simulink model "BLDC_sims"  (R2024b)
settings: Solver=ode23s  StartTime=0.0  StopTime=3  MinStep=5e-5  RelTol=1e-3
values from neighbouring files (symbols this model uses):
  b_eq = b_l*(1/r)^2+b_m    (= 2.36823386114e-05)    [Parametros.m]
  c_pitch = cos(pitch)    [Parametros.m]
  J_eq = J_l*(1/r)^2+J_m    (= 7.12145792242e-06)    [Parametros.m]
  K_e = 0.0217    [Parametros.m]
  k_l = m*g*l_cm+m_l*g*l_l    (= 5.05042475)    [Parametros.m]
  K_t = 21.7e-3    (= 0.0217)    [Parametros.m]
  Kd_m = J_eq*n*w_pos    (= 0.0142429158448)    [Parametros.m]
  ke_int = w_obs^3    (= 125000000000)    [Parametros.m]
  ke_tita = w_obs*3    (= 15000)    [Parametros.m]
  ke_w = 3*w_obs^2    (= 75000000)    [Parametros.m]
  Ki_m = J_eq*w_pos^3    (= 3646.18645628)    [Parametros.m]
  Kp_m = J_eq*n*w_pos^2    (= 11.3943326759)    [Parametros.m]
  L_s = 0.113e-3    (= 0.000113)    [Parametros.m]
  p = 7    [Parametros.m]
  p_i = -3200    [Parametros.m]
  r = 156    [Parametros.m]
  R_s = 0.196    [Parametros.m]
  s_pitch = sin(pitch)    [Parametros.m]
  s_roll = sin(roll)    [Parametros.m]
  U_d = 18    [Parametros.m]
libraries: nesl_utility x17, ee_lib x13, fl_lib x9, sdl_lib x1, spsPWMGeneratorDCDCLib x1
settings Model: Creator=ribei  LastModifiedBy=ribei
settings DataIOCC: ExternalInput=q_vel  LoadExternalInput=on

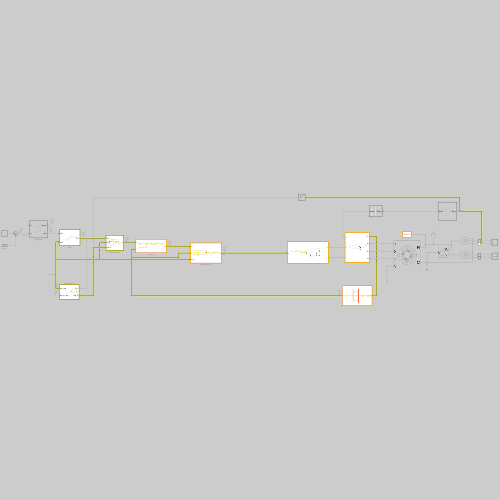
[thumbnail: Simulink's stored preview of the top-level diagram]
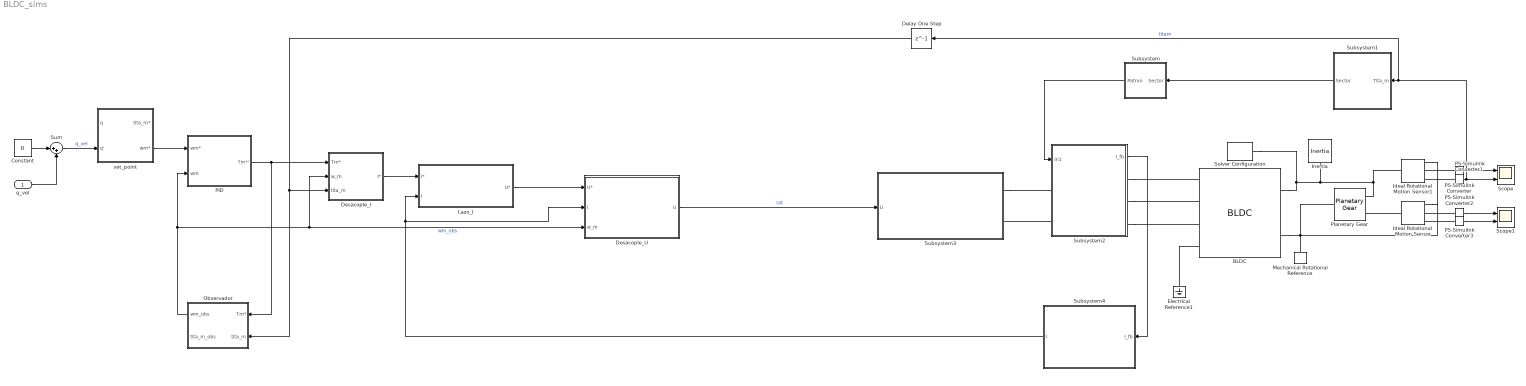
== system BLDC_sims ==
  q_vel : Inport
  BLDC : ee_lib/Electromechanical/Permanent Magnet/BLDC  port_option=ee.enum.threePhasePort.expanded  rotor_param=ee.enum.pmsm.backemf.trapezoidflux  pm_flux_linkage=0.0021 Wb  theta_constant=pi / 12 rad  emf_max=9.6 V  w_meas=600 rpm  DphiDtheta_tab=[0, -.1528, -.1528, .1528, .1528, 0] Wb/rad  back_emf_tab=[0, -9.6, -9.6, 9.6, 9.6, 0] V  rotor_angle_tab=[0, 7.5, 22.5, 37.5, 52.5, 60] deg  nPolePairs=7  axes_param=ee.enum.rotorangle.daxis  winding_type=ee.enum.electromech.statorconfiguration.wye  stator_param=ee.enum.statorparam.LdLqL0  machine_param=ee.enum.dqparameterization.constant  Ld=0.113 H  Lq=0.113 H  idVec=[-200, 0, 200] A  iqVec=[-200, 0, 200] A  LdMatrix=0.00022 * ones(3, 3) H  LqMatrix=0.00022 * ones(3, 3) H  L0=0.113 H  Ls=0.0002 H  Lm=0 H  Ms=0.00002 H  Rs=0.196 Ohm  zero_sequence=ee.enum.park.zerosequence.include  loss_param=ee.enum.ironloss.none  losses_oc=[0, 0, 0] W  losses_sc=[0, 0, 0] W  f_losses=60 Hz  Isc_losses=95 A  J=2.3e-6 kg*m^2  lam=1.184e-05 N*m*s/rad  i_d_specify=off  i_d_priority=None  i_d=0 A  i_d_nominal_specify=off  i_d_nominal_value=1  i_d_nominal_unit=A  i_q_specify=off  i_q_priority=None  i_q=0 A  i_q_nominal_specify=off  i_q_nominal_value=1  i_q_nominal_unit=A  torque_specify=off  torque_priority=None  torque=0 N*m  torque_nominal_specify=on  torque_nominal_value=0.105  torque_nominal_unit=N*m  angular_velocity_specify=off  angular_velocity_priority=High  angular_velocity=0 rpm  angular_velocity_nominal_specify=on  angular_velocity_nominal_value=6890  angular_velocity_nominal_unit=rpm  angular_position_specify=off  angular_position_priority=High  angular_position=0 deg  angular_position_nominal_specify=off  angular_position_nominal_value=1  angular_position_nominal_unit=deg  alpha=3.93e-3 1/K  alpha_flux=-0.001 1/K  Tmeas=298.15 K  stator_thermal_mass=100 J/K  rotor_thermal_mass=200 J/K  Rm_percent_rotor=90  Rd_percent_rotor=30  temperatureA_specify=off  temperatureA_priority=High  temperatureA=25 degC  temperatureA_nominal_specify=off  temperatureA_nominal_value=1  temperatureA_nominal_unit=degC  temperatureB_specify=off  temperatureB_priority=High  temperatureB=25 degC  temperatureB_nominal_specify=off  temperatureB_nominal_value=1  temperatureB_nominal_unit=degC  temperatureC_specify=off  temperatureC_priority=High  temperatureC=25 degC  temperatureC_nominal_specify=off  temperatureC_nominal_value=1  temperatureC_nominal_unit=degC  temperatureR_specify=off  temperatureR_priority=High  temperatureR=25 degC  temperatureR_nominal_specify=off  temperatureR_nominal_value=1  temperatureR_nominal_unit=degC
      settings: InternalSimscapePortConfiguration="{\"Bottom\":[],\"Left\":[{\"id\":\"a\",\"label\":\"a\",\"type\":\"foundation.electrical.electrical\"},{\"id\":\"b\",\"label\":\"b\",\"type\":\"foundation.electrical.electrical\"},{\"id\":\"c\",\"label\":\"c\",\"type\":\"foundation.electrical.electrical\"},{\"id\":\"n\",\"label\":\"n\",\"type\":\"foundation.electrical.electrical\"}],\"Right\":[{\"id\":\"R\",\"label\":\"R\",\"type\":\"foundation.mechanical.rotational.rotational\"},{\"id\":\"C\",\"label\":\"C\",\"type\":\"foundation.mechanical.rotational.rotational\"}],\"Top\":[]}"
  Constant : Constant  Value=0
  Delay One Step : Delay  DelayLength=1
  Desacople_I : Subsystem
  Desacople_U : Subsystem
  Electrical Reference1 : fl_lib/Electrical/Electrical Elements/Electrical Reference
  Ideal Rotational Motion Sensor : fl_lib/Mechanical/Mechanical Sensors/Ideal Rotational Motion Sensor  reference=foundation.enum.MeasurementReference.difference  acceleration_port=false  velocity_port=true  position_port=true  wrap_angle=false  offset=0 rad
  Ideal Rotational Motion Sensor1 : fl_lib/Mechanical/Mechanical Sensors/Ideal Rotational Motion Sensor  reference=foundation.enum.MeasurementReference.difference  acceleration_port=false  velocity_port=true  position_port=true  wrap_angle=false  offset=0 rad
  Inertia : fl_lib/Mechanical/Rotational Elements/Inertia  inertia=0.1173 kg*m^2  num_ports=foundation.enum.numPorts2.one  w_specify=off  w_priority=High  w=0 rad/s  w_nominal_specify=off  w_nominal_value=1  w_nominal_unit=rad/s  t_specify=off  t_priority=None  t=0 N*m  t_nominal_specify=off  t_nominal_value=1  t_nominal_unit=N*m
  Lazo_I : Subsystem
  Mechanical Rotational Reference : fl_lib/Mechanical/Rotational Elements/Mechanical Rotational Reference
  Observador : Subsystem
  PID : Subsystem
  PS-Simulink Converter{,1..3} (4 alike) : nesl_utility/PS-Simulink Converter  PhysicalDomain=network_engine_domain  SubClassName=ps_output  LeftPortType=input  RightPortType=output  PseudoPeriodic=off  Frequencies=[]  VectorFormat=inherit  Unit=inherit  AffineConversion=off
  Planetary Gear : sdl_lib/Gears/Planetary Gear  rs_ratio=156  friction_model=sdl.enum.gear_friction.none  efficiency=[.96, .98]  temperature_TLU=[280, 300, 320] K  efficiency_sp_TLU=[.95, .9, .85]  efficiency_rp_TLU=[.95, .9, .85]  pwr_thr=[.001, .001] W  mu_visc=[0, 0] N*m*s/rad  model_inertia=simscape.enum.onoff.off  sun_inertia=0.001 kg*m^2  ring_inertia=0.001 kg*m^2  carrier_inertia=0.001 kg*m^2  carrier_radius=0.01 m  planet_inertia=0.001 kg*m^2  planet_mass=0.001 kg  thermal_mass=50 J/K  T_init=300 K
  Scope : Scope  NumInputPorts=2
  Scope1 : Scope  NumInputPorts=2
  Solver Configuration : nesl_utility/Solver Configuration  PhysicalDomain=network_engine_domain  SubClassName=solver  LeftPortType=input  RightPortType=generic  Tones=[]  Harmonics=[]  SimulateNoise=off  Profile=off  UseLocalSampling=off  EnableSwitchedLinearOptims=on  FrequencyDomain=off  UseCCode=off  RelTol=0.001  AbsTol=0.001  MinStep=1e-09  ToWorkspace=off  RevertToSquareIcSolve=off  NumHomotopyIterations=100  PhasorMode=off  PhasorModeNumHarmonics=1  ConsistencySolver=NEWTON_XTOL_AFTER_FTOL  IndexReductionMethod=DerivativeReplacement  DoDC=off  ResidualTolerance=1e-09  ConsistencyTolSource=GLOBAL  ConsistencyAbsTol=0.001  ConsistencyRelTol=0.001  ConsistencyTolFactor=1e-9  UseLocalSolver=on  LocalSolverChoice=NE_BACKWARD_EULER_ADVANCER  ResolveIndetEquations=off  FunctionEvalNumThread=1  LocalSolverSampleTime=5e-5  DoFixedCost=on  MaxNonlinIter=3  MaxModeIter=2  ComputeImpulses=off  ImpulseIterations=2  LinearAlgebra=auto  LinearAlgebraNumThread=0  EquationFormulation=NE_TIME_EF  DelaysMemoryBudget=1024  AutomaticFiltering=on  FilteringTimeConstant=0.001  PartitionStorageMethod=AS_NEEDED  PartitionMemoryBudget=1024  PartitionMethod=ROBUST  MultibodyUseLocalSolver=off  MultibodyLocalSolverChoice=ODE1  MultibodyLocalSolverSampleTime=0.001
  Subsystem : Subsystem
  Subsystem1 : Subsystem
  Subsystem2 : Subsystem
  Subsystem3 : Subsystem
  Subsystem4 : Subsystem
  Sum : Sum  Inputs=|++
  set_point : Subsystem
  wires:
  Subsystem1/1(Sector) -> Subsystem/1(Sector)
  Subsystem/1(Patron) -> Subsystem2/1(In1)
  PS-Simulink Converter/1 -> Scope/1
  PS-Simulink Converter2/1 -> Scope1/1
  PS-Simulink Converter3/1 -> Scope1/2
  Subsystem4/1(I) -> Desacople_U/2(I), Lazo_I/2(I)
  Observador/1(wm_obs) -> PID/2(wm), Desacople_I/2(w_m), Desacople_U/3(w_m)  "wm_obs"
  PS-Simulink Converter1/1 -> Delay One Step/1, Subsystem1/1(Tita_m), Scope/2  "titam"
  set_point/2(wm*) -> PID/1(wm*)
  Lazo_I/1(U*) -> Desacople_U/1(U*)
  Constant/1 -> Sum/1
  Sum/1 -> set_point/2(q')  "q_vel"
  PID/1(Tm*') -> Observador/1(Tm*), Desacople_I/1(Tm*)
  q_vel/1 -> Sum/2
  Desacople_I/1(I*) -> Lazo_I/1(I*)
  Subsystem2/1(I_fb) -> Subsystem4/1(I_fb)
  Desacople_U/1(U) -> Subsystem3/1(U)  "Ud"
  Delay One Step/1 -> Observador/2(tita_m), Desacople_I/3(tita_m)
  connections:
  BLDC/RConn1 -- Solver Configuration/RConn1 -- Ideal Rotational Motion Sensor1/LConn1 -- Planetary Gear/RConn1 -- Inertia/LConn1
  BLDC/RConn2 -- Planetary Gear/LConn1 -- Mechanical Rotational Reference/LConn1 -- Ideal Rotational Motion Sensor1/RConn1 -- Ideal Rotational Motion Sensor/RConn1
  Ideal Rotational Motion Sensor/LConn1 -- Planetary Gear/RConn2
  PS-Simulink Converter/LConn1 -- Ideal Rotational Motion Sensor1/RConn2
  PS-Simulink Converter1/LConn1 -- Ideal Rotational Motion Sensor1/RConn3
  PS-Simulink Converter2/LConn1 -- Ideal Rotational Motion Sensor/RConn2
  PS-Simulink Converter3/LConn1 -- Ideal Rotational Motion Sensor/RConn3
  Subsystem2/RConn1 -- BLDC/LConn1
  Subsystem2/RConn2 -- BLDC/LConn2
  Subsystem2/RConn3 -- BLDC/LConn3
  Subsystem3/RConn1 -- Subsystem2/LConn1
  Subsystem2/LConn2 -- Subsystem3/RConn2
  BLDC/LConn4 -- Electrical Reference1/LConn1

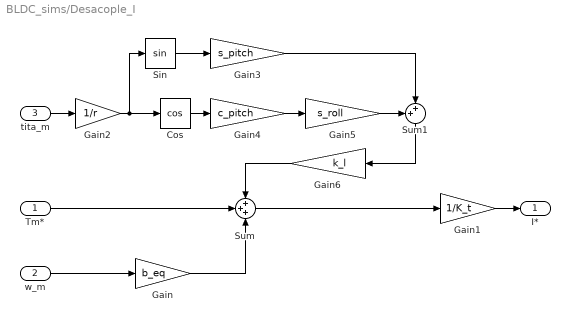
== system BLDC_sims/Desacople_I ==
  Tm* : Inport
  w_m : Inport  Port=2
  tita_m : Inport  Port=3
  Cos : Trigonometry  Operator=cos
  Gain : Gain  Gain=b_eq
  Gain1 : Gain  Gain=1/K_t
  Gain2 : Gain  Gain=1/r
  Gain3 : Gain  Gain=s_pitch
  Gain4 : Gain  Gain=c_pitch
  Gain5 : Gain  Gain=s_roll
  Gain6 : Gain  Gain=k_l
  Sin : Trigonometry
  Sum : Sum  Inputs=+++
  Sum1 : Sum  Inputs=++|
  I* : Outport
  wires:
  w_m/1 -> Gain/1
  Gain/1 -> Sum/3
  Sum/1 -> Gain1/1
  Gain1/1 -> I*/1
  Gain2/1 -> Cos/1, Sin/1
  tita_m/1 -> Gain2/1
  Cos/1 -> Gain4/1
  Sin/1 -> Gain3/1
  Sum1/1 -> Gain6/1
  Gain4/1 -> Gain5/1
  Gain5/1 -> Sum1/1
  Gain3/1 -> Sum1/2
  Gain6/1 -> Sum/1
  Tm*/1 -> Sum/2

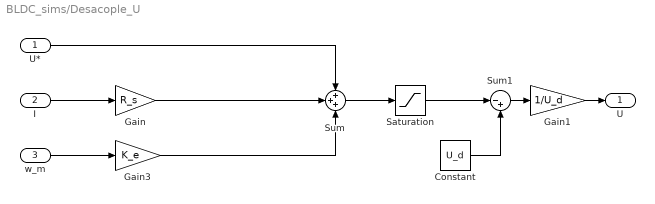
== system BLDC_sims/Desacople_U ==
  U* : Inport
  I : Inport  Port=2
  w_m : Inport  Port=3
  Constant : Constant  Value=U_d
  Gain : Gain  Gain=R_s
  Gain1 : Gain  Gain=1/U_d
  Gain3 : Gain  Gain=K_e
  Saturation : Saturate  UpperLimit=18  LowerLimit=-18
  Sum : Sum  Inputs=+++
  Sum1 : Sum  Inputs=|-+
  U : Outport
  wires:
  I/1 -> Gain/1
  w_m/1 -> Gain3/1
  Gain/1 -> Sum/2
  U*/1 -> Sum/1
  Gain3/1 -> Sum/3
  Sum/1 -> Saturation/1
  Saturation/1 -> Sum1/1
  Constant/1 -> Sum1/2
  Sum1/1 -> Gain1/1
  Gain1/1 -> U/1

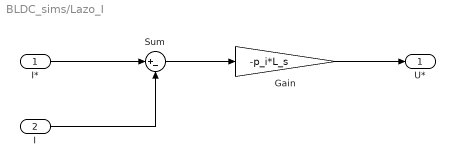
== system BLDC_sims/Lazo_I ==
  I* : Inport
  I : Inport  Port=2
  Gain : Gain  Gain=-p_i*L_s
  Sum : Sum  Inputs=|+-
  U* : Outport
  wires:
  I*/1 -> Sum/1
  I/1 -> Sum/2
  Gain/1 -> U*/1
  Sum/1 -> Gain/1

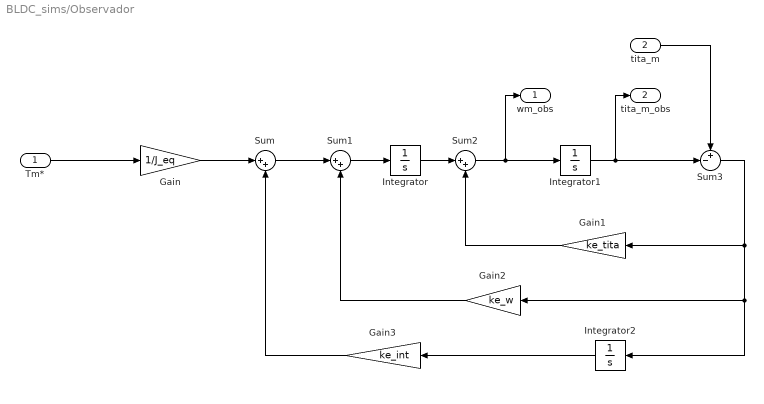
== system BLDC_sims/Observador ==
  Tm* : Inport
  tita_m : Inport  Port=2
  Gain : Gain  Gain=1/J_eq
  Gain1 : Gain  Gain=ke_tita
  Gain2 : Gain  Gain=ke_w
  Gain3 : Gain  Gain=ke_int
  Integrator : Integrator
  Integrator1 : Integrator  InitialCondition=pi/6
  Integrator2 : Integrator
  Sum : Sum  Inputs=|++
  Sum1 : Sum  Inputs=|++
  Sum2 : Sum  Inputs=|++
  Sum3 : Sum  Inputs=+-|
  wm_obs : Outport
  tita_m_obs : Outport  Port=2
  wires:
  Tm*/1 -> Gain/1
  Gain/1 -> Sum/1
  Sum/1 -> Sum1/1
  Sum1/1 -> Integrator/1
  Integrator/1 -> Sum2/1
  Sum2/1 -> wm_obs/1, Integrator1/1
  Integrator1/1 -> tita_m_obs/1, Sum3/2
  tita_m/1 -> Sum3/1
  Sum3/1 -> Gain1/1, Gain2/1, Integrator2/1
  Gain1/1 -> Sum2/2
  Gain2/1 -> Sum1/2
  Integrator2/1 -> Gain3/1
  Gain3/1 -> Sum/2

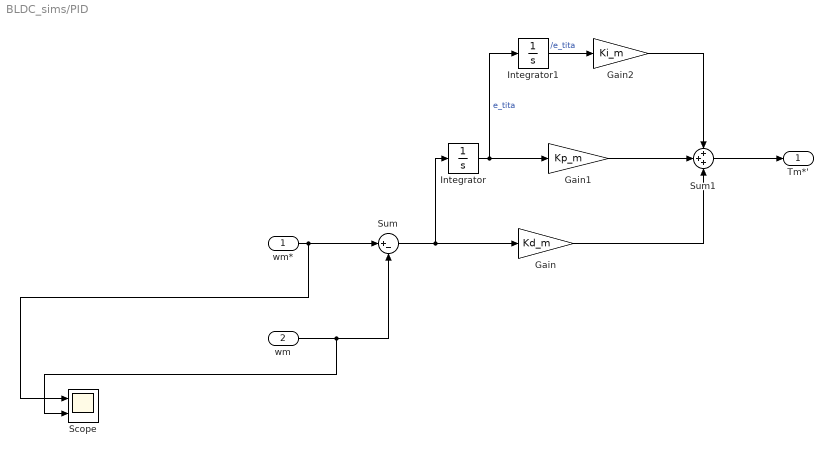
== system BLDC_sims/PID ==
  wm* : Inport
  wm : Inport  Port=2
  Gain : Gain  Gain=Kd_m
  Gain1 : Gain  Gain=Kp_m
  Gain2 : Gain  Gain=Ki_m
  Integrator : Integrator
  Integrator1 : Integrator
  Scope : Scope  NumInputPorts=2
  Sum : Sum  Inputs=|+-
  Sum1 : Sum  Inputs=+++
  Tm*' : Outport
  wires:
  Gain2/1 -> Sum1/1
  Gain/1 -> Sum1/3
  Gain1/1 -> Sum1/2
  Sum1/1 -> Tm*'/1
  wm/1 -> Scope/2, Sum/2
  Integrator/1 -> Gain1/1, Integrator1/1  "e_tita"
  Integrator1/1 -> Gain2/1  "/e_tita"
  wm*/1 -> Scope/1, Sum/1
  Sum/1 -> Gain/1, Integrator/1

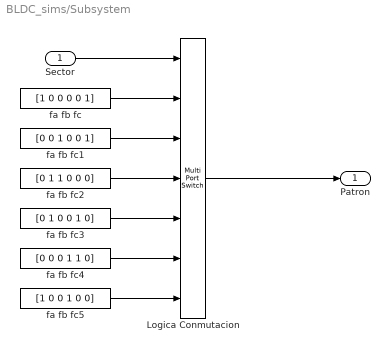
== system BLDC_sims/Subsystem ==
  Sector : Inport
  Logica Conmutacion : MultiPortSwitch  Inputs=6  DiagnosticForDefault=None  SaturateOnIntegerOverflow=off  InputSameDT=off
  fa fb fc : Constant  Value=[1 0 0 0 0 1]
  fa fb fc1 : Constant  Value=[0 0 1 0 0 1]
  fa fb fc2 : Constant  Value=[0 1 1 0 0 0]
  fa fb fc3 : Constant  Value=[0 1 0 0 1 0]
  fa fb fc4 : Constant  Value=[0 0 0 1 1 0]
  fa fb fc5 : Constant  Value=[1 0 0 1 0 0]
  Patron : Outport
  wires:
  fa fb fc3/1 -> Logica Conmutacion/5
  fa fb fc4/1 -> Logica Conmutacion/6
  fa fb fc1/1 -> Logica Conmutacion/3
  Sector/1 -> Logica Conmutacion/1
  Logica Conmutacion/1 -> Patron/1
  fa fb fc/1 -> Logica Conmutacion/2
  fa fb fc5/1 -> Logica Conmutacion/7
  fa fb fc2/1 -> Logica Conmutacion/4

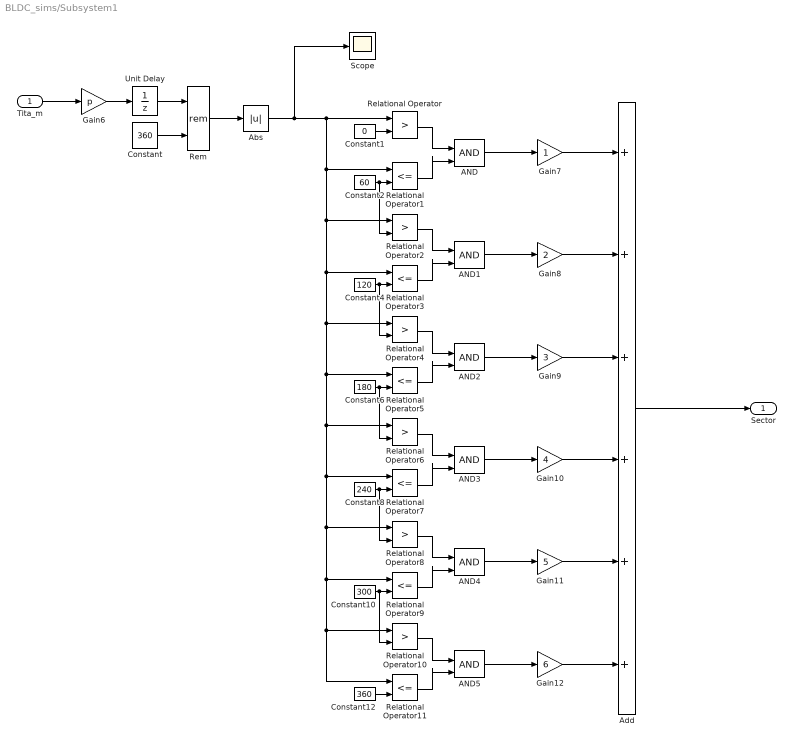
== system BLDC_sims/Subsystem1 ==
  Tita_m : Inport
  AND{,1..5} (6 alike) : Logic  IconShape=distinctive  AllPortsSameDT=off  OutDataTypeStr=boolean
  Abs : Abs  SaturateOnIntegerOverflow=off
  Add : Sum  Inputs=++++++
  Constant : Constant  Value=360
  Constant1 : Constant  Value=0
  Constant10 : Constant  Value=300
  Constant12 : Constant  Value=360
  Constant2 : Constant  Value=60
  Constant4 : Constant  Value=120
  Constant6 : Constant  Value=180
  Constant8 : Constant  Value=240
  Gain10 : Gain  Gain=4
  Gain11 : Gain  Gain=5
  Gain12 : Gain  Gain=6
  Gain6 : Gain  Gain=p
  Gain7 : Gain
  Gain8 : Gain  Gain=2
  Gain9 : Gain  Gain=3
  Relational Operator{,2,4,6,8,10} (6 alike) : RelationalOperator  Operator=>  OutDataTypeStr=boolean  RndMeth=Simplest  InputSameDT=off
  Relational Operator{1,3,5,7,9,11} (6 alike) : RelationalOperator  Operator=<=  OutDataTypeStr=boolean  RndMeth=Simplest  InputSameDT=off
  Rem : Math  Operator=rem
  Scope : Scope
  Unit Delay : UnitDelay  SampleTime=0.001  HasFrameUpgradeWarning=on
  Sector : Outport
  wires:
  Rem/1 -> Abs/1
  AND4/1 -> Gain11/1
  AND1/1 -> Gain8/1
  Relational Operator4/1 -> AND2/1
  Add/1 -> Sector/1
  Gain10/1 -> Add/4
  Relational Operator8/1 -> AND4/1
  Relational Operator3/1 -> AND1/2
  Relational Operator2/1 -> AND1/1
  Gain9/1 -> Add/3
  Constant4/1 -> Relational Operator4/2, Relational Operator3/2
  Constant6/1 -> Relational Operator6/2, Relational Operator5/2
  Gain11/1 -> Add/5
  Constant2/1 -> Relational Operator2/2, Relational Operator1/2
  AND2/1 -> Gain9/1
  Gain7/1 -> Add/1
  Relational Operator5/1 -> AND2/2
  Constant10/1 -> Relational Operator10/2, Relational Operator9/2
  AND/1 -> Gain7/1
  Constant1/1 -> Relational Operator/2
  Relational Operator/1 -> AND/1
  Constant/1 -> Rem/2
  Relational Operator11/1 -> AND5/2
  Constant12/1 -> Relational Operator11/2
  Relational Operator10/1 -> AND5/1
  AND5/1 -> Gain12/1
  Relational Operator9/1 -> AND4/2
  Unit Delay/1 -> Rem/1
  Gain12/1 -> Add/6
  Gain6/1 -> Unit Delay/1
  Tita_m/1 -> Gain6/1
  Constant8/1 -> Relational Operator8/2, Relational Operator7/2
  Relational Operator1/1 -> AND/2
  Relational Operator7/1 -> AND3/2
  AND3/1 -> Gain10/1
  Relational Operator6/1 -> AND3/1
  Gain8/1 -> Add/2
  Abs/1 -> Scope/1, Relational Operator/1, Relational Operator1/1, Relational Operator2/1, Relational Operator3/1, Relational Operator4/1, Relational Operator5/1, Relational Operator6/1, Relational Operator7/1, Relational Operator8/1, Relational Operator9/1, Relational Operator10/1, Relational Operator11/1

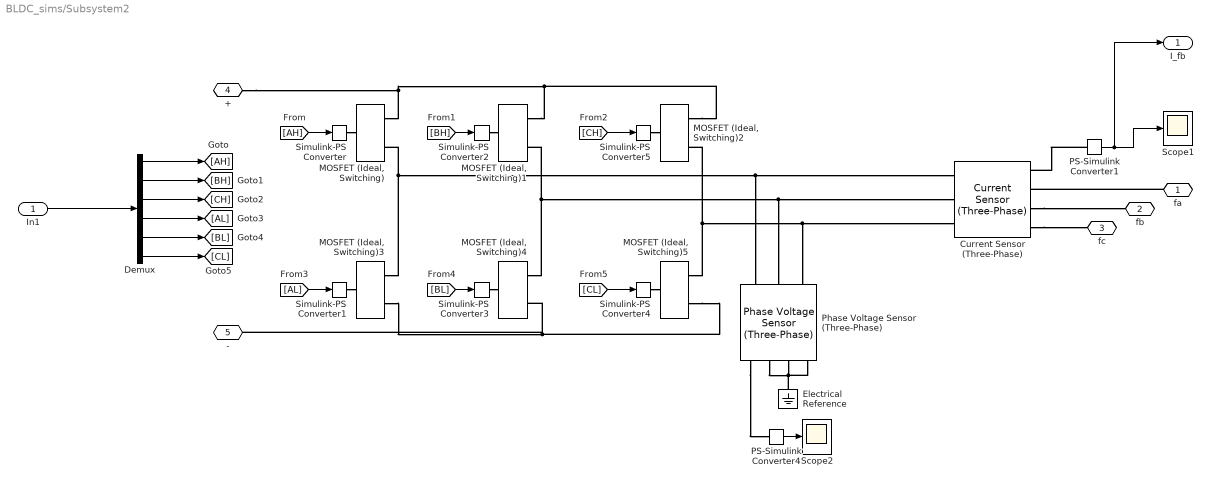
== system BLDC_sims/Subsystem2 ==
  In1 : Inport
  Current Sensor (Three-Phase) : ee_lib/Sensors & Transducers/Current Sensor (Three-Phase)
      settings: InternalSimscapePortConfiguration="{\"Bottom\":[],\"Left\":[{\"id\":\"a1\",\"label\":\"a1\",\"type\":\"foundation.electrical.electrical\"},{\"id\":\"b1\",\"label\":\"b1\",\"type\":\"foundation.electrical.electrical\"},{\"id\":\"c1\",\"label\":\"c1\",\"type\":\"foundation.electrical.electrical\"}],\"Right\":[{\"id\":\"I_output\",\"label\":\"I\",\"type\":\"output\"},{\"id\":\"a2\",\"label\":\"a2\",\"type\":\"foundation.electrical.electrical\"},{\"id\":\"b2\",\"label\":\"b2\",\"type\":\"foundation.electrical.electrical\"},{\"id\":\"c2\",\"label\":\"c2\",\"type\":\"foundation.electrical.electrical\"}],\"Top\":[]}"
  Demux : Demux  Outputs=6
  Electrical Reference : fl_lib/Electrical/Electrical Elements/Electrical Reference
  MOSFET (Ideal, Switching){,1..5} (6 alike) : ee_lib/Semiconductors & Converters/MOSFET (Ideal, Switching)  port_option=ee.enum.controlport.ps  Rds=0.01 Ohm  Goff=1e-6 1/Ohm  Vth=2 V  diode_param=ee.enum.semiconductors.protectionDiode.nodynamics  diode_Vf=0.8 V  diode_Ron=0.001 Ohm  diode_Goff=1e-5 1/Ohm  diode_C=50e-9 F  diode_iRM=-235 A  diode_iF=300 A  diode_idot=-50 A/us  diode_trr_param=ee.enum.converters.diodeReverseParam.trr_factor  diode_trr_factor=3  diode_trr=15 us  diode_Qrr=1500 s*uA  ids_specify=off  ids_priority=None  ids=0 A  ids_nominal_specify=off  ids_nominal_value=1  ids_nominal_unit=A  vds_specify=off  vds_priority=None  vds=0 V  vds_nominal_specify=off  vds_nominal_value=1  vds_nominal_unit=V  vgs_specify=off  vgs_priority=None  vgs=0 V  vgs_nominal_specify=off  vgs_nominal_value=1  vgs_nominal_unit=V  thermal_loss_option=ee.enum.converters.thermalLossOption.constantvalues  Von_data=[0, 1.8, 3.2, 6, 10, 16; 0, 2, 5.5, 9.5, 15, 25] V  Tj=[298.15, 448.15] K  Iout_data=[0, 20, 40, 60, 80, 100] A  Eon_data=[0, 55.04, 124.57, 235.53, 362.12; 0, 71.25, 161.25, 304.88, 468.75] * 1e-6 J  Eoff_data=[0, 18, 30, 56.1, 76.5; 0, 22.5, 37.5, 70.13, 95.63] * 1e-6 J  Eon_data_3D=[zeros(2, 5, 3)] J  Eoff_data_3D=[zeros(2, 5, 3)] J  Tj_loss=[298.15, 448.15] K  Iout_data_loss=[0, 10, 20, 30, 40] A  tabulateWithVds=false  Vds_loss=[0, 150, 300] V  Eon_scalar=22.86e-3 J  Eoff_scalar=17.14e-3 J  Voff=300 V  Iout_scalar=600 A  useCurrentFromPreviousCycle=false  useVoltageFromPreviousCycle=false  diodeModelType=ee.enum.converters.diodeModelType.pwl  diodeTableType=ee.enum.diode.tableType.IfMat  diode_ReverseIVType=ee.enum.diode.diodeReverseIV.constant  diode_IfMat=[.07, .12, .19, 1.75, 4.24, 7.32, 11.2; .16, .3, .72, 2.14, 4.02, 6.35, 9.12] A  diode_VfMat=[.9, 1.15, 1.25, 1.5, 1.75, 2.17, 2.6, 2.85; .58, .68, .75, 1.1, 1.38, 1.77, 2.27, 2.7] V  diode_TjVec=[25, 125] degC  diode_VfVec=[.5, .7, .9, 1.3, 1.7, 2.1, 2.5] V  diode_IfVec=[.1, .2, .5, 1, 2, 4, 7, 10] A  diode_IrMat=[1e-06, 2e-06, 5e-06, 1e-05, 2.5e-05, 5e-05, .0001; 2e-06, 5e-06, 1e-05, 4e-05, 8e-05, .0002, .0005] A  diode_VrMat=[10, 100, 200, 250, 300, 325, 350; 10, 70, 160, 220, 270, 300, 320] V  diode_VrVec=[10, 20, 40, 50, 70, 80, 100] V  diode_IrVec=[1e-06, 2e-06, 5e-06, 1e-05, 2e-05, 5e-05, .0001] A  diode_Vr=-600 V  diode_Ls=150 nH  diode_Erec=0.03 J  diode_rec_loss_model=ee.enum.diode.reverseRecoveryModel.fixed  diode_ErecVal=0 J  diode_scaleWithIandV=true  diode_ErecMat=zeros(2, 3) J  diode_TjrecVec=[298.15, 398.15] K  diode_IfrecVec=[.1, 1, 10] A  diode_IrecVal=10 A  diode_VrecVal=10 V  diode_tFilter=1 / 1000 / 100 s  separateThermalPortForDiode=false  thermal_network_parameterization=ee.enum.thermalNetworkTopology.external  Rth=[.03, .2] K/W  Rth_Cauer=[.03, .1, .2] K/W  Rth_Foster=[.08, .14, .22, .16] K/W  thermal_mass_parameterization=ee.enum.thermalNetwork.timeconstant  thermal_mass=[3, 25] J/K  thermal_mass_Cauer=[3, 10, 25] J/K  thermal_mass_Foster=[.001, .005, .05, .5] J/K  thermal_time_constant=[.1, 5] s  thermal_time_constant_Cauer=[.1, 1, 5] s  thermal_time_constant_Foster=[7e-05, .0007, .01, .08] s  thermal_mass_initial_temperatures=[25, 25] degC  thermal_mass_initial_temperatures_Cauer=[25, 25, 25] degC  junction_thermal_mass=0.1 J/K  Tvec_initial_Foster=[25, 25, 25, 25] degC  RthDiode=[.03, .2] K/W  RthCauerDiode=[.03, .1, .2] K/W  RthFosterDiode=[.03, .2] K/W  thermalMassDiode=[3, 25] J/K  thermalMassCauerDiode=[3, 10, 25] J/K  thermalMassFosterDiode=[33, 50] J/K  thermalTauDiode=[.1, 5] s  thermalTauCauerDiode=[.1, 1, 5] s  thermalTauFosterDiode=[1, 10] s  thermalMassInitTempDiode=[25, 25] degC  thermalMassInitTempCauerDiode=[25, 25, 25] degC  junctionthermalMassDiode=0.1 J/K  TVecInitialFosterDiode=[25, 25, 25, 25] degC  no_thermal_network=0  mosfet_junction_temperature_specify=off  mosfet_junction_temperature_priority=None  mosfet_junction_temperature=25 degC  mosfet_junction_temperature_nominal_specify=off  mosfet_junction_temperature_nominal_value=1  mosfet_junction_temperature_nominal_unit=degC  diode_junction_temperature_specify=off  diode_junction_temperature_priority=None  diode_junction_temperature=25 degC  diode_junction_temperature_nominal_specify=off  diode_junction_temperature_nominal_value=1  diode_junction_temperature_nominal_unit=degC  Qj_specify=off  Qj_priority=None  Qj=0 W  Qj_nominal_specify=off  Qj_nominal_value=1  Qj_nominal_unit=W  accumulatedSwitchingLosses_specify=off  accumulatedSwitchingLosses_priority=None  accumulatedSwitchingLosses=0 J
  PS-Simulink Converter1 : nesl_utility/PS-Simulink Converter  PhysicalDomain=network_engine_domain  SubClassName=ps_output  LeftPortType=input  RightPortType=output  PseudoPeriodic=off  Frequencies=[]  VectorFormat=inherit  Unit=inherit  AffineConversion=off
  PS-Simulink Converter4 : nesl_utility/PS-Simulink Converter  PhysicalDomain=network_engine_domain  SubClassName=ps_output  LeftPortType=input  RightPortType=output  PseudoPeriodic=off  Frequencies=[]  VectorFormat=inherit  Unit=inherit  AffineConversion=off
  Phase Voltage Sensor (Three-Phase) : ee_lib/Sensors & Transducers/Phase Voltage Sensor (Three-Phase)
      settings: InternalSimscapePortConfiguration="{\"Bottom\":[],\"Left\":[{\"id\":\"a1\",\"label\":\"a1\",\"type\":\"foundation.electrical.electrical\"},{\"id\":\"b1\",\"label\":\"b1\",\"type\":\"foundation.electrical.electrical\"},{\"id\":\"c1\",\"label\":\"c1\",\"type\":\"foundation.electrical.electrical\"}],\"Right\":[{\"id\":\"V_output\",\"label\":\"V\",\"type\":\"output\"},{\"id\":\"a2\",\"label\":\"a2\",\"type\":\"foundation.electrical.electrical\"},{\"id\":\"b2\",\"label\":\"b2\",\"type\":\"foundation.electrical.electrical\"},{\"id\":\"c2\",\"label\":\"c2\",\"type\":\"foundation.electrical.electrical\"}],\"Top\":[]}"
  Scope1 : Scope
  Scope2 : Scope
  Simulink-PS Converter{,1..5} (6 alike) : nesl_utility/Simulink-PS Converter  PhysicalDomain=network_engine_domain  SubClassName=ps_input  LeftPortType=input  RightPortType=output  PseudoPeriodic=off  Frequencies=[]  NoiseDistribution=none  NoiseParameters=[]  Unit=1  AffineConversion=off  FilteringAndDerivatives=provide  SimscapeFilterOrder=1  InputFilterTimeConstant=0.001  UdotUserProvided=0
  fa : PMIOPort  Side=Right
  fb : PMIOPort  Port=2  Side=Right
  fc : PMIOPort  Port=3  Side=Right
  + : PMIOPort  Port=4  Side=Left
  - : PMIOPort  Port=5  Side=Left
  I_fb : Outport
  wires:
  In1/1 -> Demux/1
  Demux/6 -> [CL]
  [BH] -> Simulink-PS Converter2/1
  Demux/1 -> [AH]
  Demux/2 -> [BH]
  Demux/3 -> [CH]
  [AH] -> Simulink-PS Converter/1
  [BL] -> Simulink-PS Converter3/1
  [AL] -> Simulink-PS Converter1/1
  Demux/5 -> [BL]
  [CL] -> Simulink-PS Converter4/1
  Demux/4 -> [AL]
  [CH] -> Simulink-PS Converter5/1
  PS-Simulink Converter4/1 -> Scope2/1
  PS-Simulink Converter1/1 -> I_fb/1, Scope1/1
  connections:
  "MOSFET (Ideal, Switching)"/RConn1 -- "MOSFET (Ideal, Switching)2"/RConn1 -- "MOSFET (Ideal, Switching)1"/RConn1 -- +/RConn1
  Simulink-PS Converter2/RConn1 -- "MOSFET (Ideal, Switching)1"/LConn1
  "MOSFET (Ideal, Switching)5"/RConn1 -- "MOSFET (Ideal, Switching)2"/RConn2 -- Phase Voltage Sensor (Three-Phase)/LConn3 -- Current Sensor (Three-Phase)/LConn3
  "MOSFET (Ideal, Switching)3"/RConn1 -- "MOSFET (Ideal, Switching)"/RConn2 -- Phase Voltage Sensor (Three-Phase)/LConn1 -- Current Sensor (Three-Phase)/LConn1
  Simulink-PS Converter1/RConn1 -- "MOSFET (Ideal, Switching)3"/LConn1
  Simulink-PS Converter5/RConn1 -- "MOSFET (Ideal, Switching)2"/LConn1
  Simulink-PS Converter4/RConn1 -- "MOSFET (Ideal, Switching)5"/LConn1
  Simulink-PS Converter3/RConn1 -- "MOSFET (Ideal, Switching)4"/LConn1
  "MOSFET (Ideal, Switching)4"/RConn1 -- "MOSFET (Ideal, Switching)1"/RConn2 -- Phase Voltage Sensor (Three-Phase)/LConn2 -- Current Sensor (Three-Phase)/LConn2
  Simulink-PS Converter/RConn1 -- "MOSFET (Ideal, Switching)"/LConn1
  "MOSFET (Ideal, Switching)5"/RConn2 -- "MOSFET (Ideal, Switching)3"/RConn2 -- -/RConn1 -- "MOSFET (Ideal, Switching)4"/RConn2
  Electrical Reference/LConn1 -- Phase Voltage Sensor (Three-Phase)/RConn2 -- Phase Voltage Sensor (Three-Phase)/RConn4 -- Phase Voltage Sensor (Three-Phase)/RConn3
  Phase Voltage Sensor (Three-Phase)/RConn1 -- PS-Simulink Converter4/LConn1
  fa/RConn1 -- Current Sensor (Three-Phase)/RConn2
  Current Sensor (Three-Phase)/RConn3 -- fb/RConn1
  Current Sensor (Three-Phase)/RConn4 -- fc/RConn1
  PS-Simulink Converter1/LConn1 -- Current Sensor (Three-Phase)/RConn1

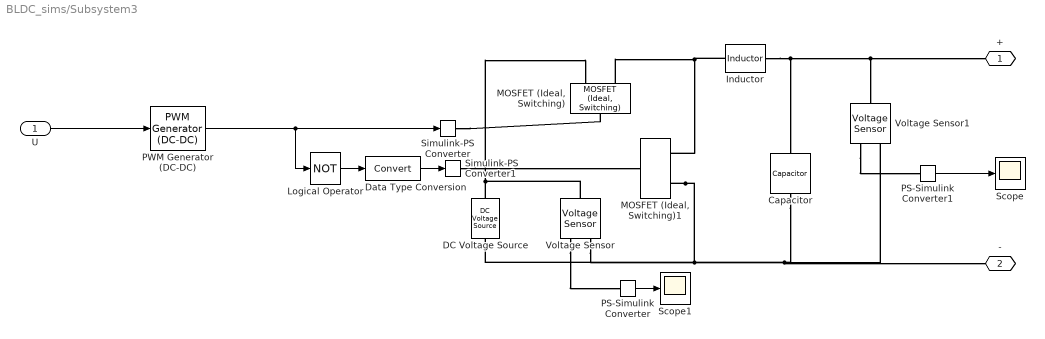
== system BLDC_sims/Subsystem3 ==
  U : Inport
  Capacitor : fl_lib/Electrical/Electrical Elements/Capacitor  c=0.01 F  r=0.2 Ohm  g=0 1/Ohm  i_specify=off  i_priority=None  i=0 A  i_nominal_specify=off  i_nominal_value=1  i_nominal_unit=A  v_specify=off  v_priority=None  v=0 V  v_nominal_specify=off  v_nominal_value=1  v_nominal_unit=V  vc_specify=off  vc_priority=High  vc=0 V  vc_nominal_specify=off  vc_nominal_value=1  vc_nominal_unit=V
  DC Voltage Source : ee_lib/Additional Components/SPICE Sources/DC Voltage Source  DC=18 V
  Data Type Conversion : DataTypeConversion  SaturateOnIntegerOverflow=off  RndMeth=Floor
  Inductor : ee_lib/Passive/Inductor  l=0.1 H  enable_L_tol=ee.enum.toleranceApplication.none  L_tol=20  tol_distribution=ee.enum.toleranceDistribution.uniform  nSigma=4  r=0.1 Ohm  g=1e-9 1/Ohm  enable_operating_limits=ee.enum.enable.no  operating_limit_action=ee.enum.passive.reportOpLim.warn  max_working_current=1 A  power_rating=1 W  fault_action=simscape.enum.assert.action.none  t_fault=1 s  i_L_specify=off  i_L_priority=High  i_L=0 A  i_L_nominal_specify=off  i_L_nominal_value=1  i_L_nominal_unit=A
  Logical Operator : Logic  Operator=NOT  AllPortsSameDT=off  OutDataTypeStr=boolean
  "MOSFET (Ideal, Switching)" : ee_lib/Semiconductors & Converters/MOSFET (Ideal, Switching)  port_option=ee.enum.controlport.ps  Rds=1e-4 Ohm  Goff=1e-6 1/Ohm  Vth=2 V  diode_param=ee.enum.semiconductors.protectionDiode.nodynamics  diode_Vf=0.1 V  diode_Ron=0.001 Ohm  diode_Goff=1e-5 1/Ohm  diode_C=50e-9 F  diode_iRM=-235 A  diode_iF=300 A  diode_idot=-50 A/us  diode_trr_param=ee.enum.converters.diodeReverseParam.trr_factor  diode_trr_factor=3  diode_trr=15 us  diode_Qrr=1500 s*uA  ids_specify=off  ids_priority=None  ids=0 A  ids_nominal_specify=off  ids_nominal_value=1  ids_nominal_unit=A  vds_specify=off  vds_priority=None  vds=0 V  vds_nominal_specify=off  vds_nominal_value=1  vds_nominal_unit=V  vgs_specify=off  vgs_priority=None  vgs=0 V  vgs_nominal_specify=off  vgs_nominal_value=1  vgs_nominal_unit=V  thermal_loss_option=ee.enum.converters.thermalLossOption.constantvalues  Von_data=[0, 1.8, 3.2, 6, 10, 16; 0, 2, 5.5, 9.5, 15, 25] V  Tj=[298.15, 448.15] K  Iout_data=[0, 20, 40, 60, 80, 100] A  Eon_data=[0, 55.04, 124.57, 235.53, 362.12; 0, 71.25, 161.25, 304.88, 468.75] * 1e-6 J  Eoff_data=[0, 18, 30, 56.1, 76.5; 0, 22.5, 37.5, 70.13, 95.63] * 1e-6 J  Eon_data_3D=[zeros(2, 5, 3)] J  Eoff_data_3D=[zeros(2, 5, 3)] J  Tj_loss=[298.15, 448.15] K  Iout_data_loss=[0, 10, 20, 30, 40] A  tabulateWithVds=false  Vds_loss=[0, 150, 300] V  Eon_scalar=22.86e-3 J  Eoff_scalar=17.14e-3 J  Voff=300 V  Iout_scalar=600 A  useCurrentFromPreviousCycle=false  useVoltageFromPreviousCycle=false  diodeModelType=ee.enum.converters.diodeModelType.pwl  diodeTableType=ee.enum.diode.tableType.IfMat  diode_ReverseIVType=ee.enum.diode.diodeReverseIV.constant  diode_IfMat=[.07, .12, .19, 1.75, 4.24, 7.32, 11.2; .16, .3, .72, 2.14, 4.02, 6.35, 9.12] A  diode_VfMat=[.9, 1.15, 1.25, 1.5, 1.75, 2.17, 2.6, 2.85; .58, .68, .75, 1.1, 1.38, 1.77, 2.27, 2.7] V  diode_TjVec=[25, 125] degC  diode_VfVec=[.5, .7, .9, 1.3, 1.7, 2.1, 2.5] V  diode_IfVec=[.1, .2, .5, 1, 2, 4, 7, 10] A  diode_IrMat=[1e-06, 2e-06, 5e-06, 1e-05, 2.5e-05, 5e-05, .0001; 2e-06, 5e-06, 1e-05, 4e-05, 8e-05, .0002, .0005] A  diode_VrMat=[10, 100, 200, 250, 300, 325, 350; 10, 70, 160, 220, 270, 300, 320] V  diode_VrVec=[10, 20, 40, 50, 70, 80, 100] V  diode_IrVec=[1e-06, 2e-06, 5e-06, 1e-05, 2e-05, 5e-05, .0001] A  diode_Vr=-600 V  diode_Ls=150 nH  diode_Erec=0.03 J  diode_rec_loss_model=ee.enum.diode.reverseRecoveryModel.fixed  diode_ErecVal=0 J  diode_scaleWithIandV=true  diode_ErecMat=zeros(2, 3) J  diode_TjrecVec=[298.15, 398.15] K  diode_IfrecVec=[.1, 1, 10] A  diode_IrecVal=10 A  diode_VrecVal=10 V  diode_tFilter=1 / 1000 / 100 s  separateThermalPortForDiode=false  thermal_network_parameterization=ee.enum.thermalNetworkTopology.external  Rth=[.03, .2] K/W  Rth_Cauer=[.03, .1, .2] K/W  Rth_Foster=[.08, .14, .22, .16] K/W  thermal_mass_parameterization=ee.enum.thermalNetwork.timeconstant  thermal_mass=[3, 25] J/K  thermal_mass_Cauer=[3, 10, 25] J/K  thermal_mass_Foster=[.001, .005, .05, .5] J/K  thermal_time_constant=[.1, 5] s  thermal_time_constant_Cauer=[.1, 1, 5] s  thermal_time_constant_Foster=[7e-05, .0007, .01, .08] s  thermal_mass_initial_temperatures=[25, 25] degC  thermal_mass_initial_temperatures_Cauer=[25, 25, 25] degC  junction_thermal_mass=0.1 J/K  Tvec_initial_Foster=[25, 25, 25, 25] degC  RthDiode=[.03, .2] K/W  RthCauerDiode=[.03, .1, .2] K/W  RthFosterDiode=[.03, .2] K/W  thermalMassDiode=[3, 25] J/K  thermalMassCauerDiode=[3, 10, 25] J/K  thermalMassFosterDiode=[33, 50] J/K  thermalTauDiode=[.1, 5] s  thermalTauCauerDiode=[.1, 1, 5] s  thermalTauFosterDiode=[1, 10] s  thermalMassInitTempDiode=[25, 25] degC  thermalMassInitTempCauerDiode=[25, 25, 25] degC  junctionthermalMassDiode=0.1 J/K  TVecInitialFosterDiode=[25, 25, 25, 25] degC  no_thermal_network=0  mosfet_junction_temperature_specify=off  mosfet_junction_temperature_priority=None  mosfet_junction_temperature=25 degC  mosfet_junction_temperature_nominal_specify=off  mosfet_junction_temperature_nominal_value=1  mosfet_junction_temperature_nominal_unit=degC  diode_junction_temperature_specify=off  diode_junction_temperature_priority=None  diode_junction_temperature=25 degC  diode_junction_temperature_nominal_specify=off  diode_junction_temperature_nominal_value=1  diode_junction_temperature_nominal_unit=degC  Qj_specify=off  Qj_priority=None  Qj=0 W  Qj_nominal_specify=off  Qj_nominal_value=1  Qj_nominal_unit=W  accumulatedSwitchingLosses_specify=off  accumulatedSwitchingLosses_priority=None  accumulatedSwitchingLosses=0 J
  "MOSFET (Ideal, Switching)1" : ee_lib/Semiconductors & Converters/MOSFET (Ideal, Switching)  port_option=ee.enum.controlport.ps  Rds=1e-4 Ohm  Goff=1e-6 1/Ohm  Vth=2 V  diode_param=ee.enum.semiconductors.protectionDiode.nodynamics  diode_Vf=0.1 V  diode_Ron=0.001 Ohm  diode_Goff=1e-5 1/Ohm  diode_C=50e-9 F  diode_iRM=-235 A  diode_iF=300 A  diode_idot=-50 A/us  diode_trr_param=ee.enum.converters.diodeReverseParam.trr_factor  diode_trr_factor=3  diode_trr=15 us  diode_Qrr=1500 s*uA  ids_specify=off  ids_priority=None  ids=0 A  ids_nominal_specify=off  ids_nominal_value=1  ids_nominal_unit=A  vds_specify=off  vds_priority=None  vds=0 V  vds_nominal_specify=off  vds_nominal_value=1  vds_nominal_unit=V  vgs_specify=off  vgs_priority=None  vgs=0 V  vgs_nominal_specify=off  vgs_nominal_value=1  vgs_nominal_unit=V  thermal_loss_option=ee.enum.converters.thermalLossOption.constantvalues  Von_data=[0, 1.8, 3.2, 6, 10, 16; 0, 2, 5.5, 9.5, 15, 25] V  Tj=[298.15, 448.15] K  Iout_data=[0, 20, 40, 60, 80, 100] A  Eon_data=[0, 55.04, 124.57, 235.53, 362.12; 0, 71.25, 161.25, 304.88, 468.75] * 1e-6 J  Eoff_data=[0, 18, 30, 56.1, 76.5; 0, 22.5, 37.5, 70.13, 95.63] * 1e-6 J  Eon_data_3D=[zeros(2, 5, 3)] J  Eoff_data_3D=[zeros(2, 5, 3)] J  Tj_loss=[298.15, 448.15] K  Iout_data_loss=[0, 10, 20, 30, 40] A  tabulateWithVds=false  Vds_loss=[0, 150, 300] V  Eon_scalar=22.86e-3 J  Eoff_scalar=17.14e-3 J  Voff=300 V  Iout_scalar=600 A  useCurrentFromPreviousCycle=false  useVoltageFromPreviousCycle=false  diodeModelType=ee.enum.converters.diodeModelType.pwl  diodeTableType=ee.enum.diode.tableType.IfMat  diode_ReverseIVType=ee.enum.diode.diodeReverseIV.constant  diode_IfMat=[.07, .12, .19, 1.75, 4.24, 7.32, 11.2; .16, .3, .72, 2.14, 4.02, 6.35, 9.12] A  diode_VfMat=[.9, 1.15, 1.25, 1.5, 1.75, 2.17, 2.6, 2.85; .58, .68, .75, 1.1, 1.38, 1.77, 2.27, 2.7] V  diode_TjVec=[25, 125] degC  diode_VfVec=[.5, .7, .9, 1.3, 1.7, 2.1, 2.5] V  diode_IfVec=[.1, .2, .5, 1, 2, 4, 7, 10] A  diode_IrMat=[1e-06, 2e-06, 5e-06, 1e-05, 2.5e-05, 5e-05, .0001; 2e-06, 5e-06, 1e-05, 4e-05, 8e-05, .0002, .0005] A  diode_VrMat=[10, 100, 200, 250, 300, 325, 350; 10, 70, 160, 220, 270, 300, 320] V  diode_VrVec=[10, 20, 40, 50, 70, 80, 100] V  diode_IrVec=[1e-06, 2e-06, 5e-06, 1e-05, 2e-05, 5e-05, .0001] A  diode_Vr=-600 V  diode_Ls=150 nH  diode_Erec=0.03 J  diode_rec_loss_model=ee.enum.diode.reverseRecoveryModel.fixed  diode_ErecVal=0 J  diode_scaleWithIandV=true  diode_ErecMat=zeros(2, 3) J  diode_TjrecVec=[298.15, 398.15] K  diode_IfrecVec=[.1, 1, 10] A  diode_IrecVal=10 A  diode_VrecVal=10 V  diode_tFilter=1 / 1000 / 100 s  separateThermalPortForDiode=false  thermal_network_parameterization=ee.enum.thermalNetworkTopology.external  Rth=[.03, .2] K/W  Rth_Cauer=[.03, .1, .2] K/W  Rth_Foster=[.08, .14, .22, .16] K/W  thermal_mass_parameterization=ee.enum.thermalNetwork.timeconstant  thermal_mass=[3, 25] J/K  thermal_mass_Cauer=[3, 10, 25] J/K  thermal_mass_Foster=[.001, .005, .05, .5] J/K  thermal_time_constant=[.1, 5] s  thermal_time_constant_Cauer=[.1, 1, 5] s  thermal_time_constant_Foster=[7e-05, .0007, .01, .08] s  thermal_mass_initial_temperatures=[25, 25] degC  thermal_mass_initial_temperatures_Cauer=[25, 25, 25] degC  junction_thermal_mass=0.1 J/K  Tvec_initial_Foster=[25, 25, 25, 25] degC  RthDiode=[.03, .2] K/W  RthCauerDiode=[.03, .1, .2] K/W  RthFosterDiode=[.03, .2] K/W  thermalMassDiode=[3, 25] J/K  thermalMassCauerDiode=[3, 10, 25] J/K  thermalMassFosterDiode=[33, 50] J/K  thermalTauDiode=[.1, 5] s  thermalTauCauerDiode=[.1, 1, 5] s  thermalTauFosterDiode=[1, 10] s  thermalMassInitTempDiode=[25, 25] degC  thermalMassInitTempCauerDiode=[25, 25, 25] degC  junctionthermalMassDiode=0.1 J/K  TVecInitialFosterDiode=[25, 25, 25, 25] degC  no_thermal_network=0  mosfet_junction_temperature_specify=off  mosfet_junction_temperature_priority=None  mosfet_junction_temperature=25 degC  mosfet_junction_temperature_nominal_specify=off  mosfet_junction_temperature_nominal_value=1  mosfet_junction_temperature_nominal_unit=degC  diode_junction_temperature_specify=off  diode_junction_temperature_priority=None  diode_junction_temperature=25 degC  diode_junction_temperature_nominal_specify=off  diode_junction_temperature_nominal_value=1  diode_junction_temperature_nominal_unit=degC  Qj_specify=off  Qj_priority=None  Qj=0 W  Qj_nominal_specify=off  Qj_nominal_value=1  Qj_nominal_unit=W  accumulatedSwitchingLosses_specify=off  accumulatedSwitchingLosses_priority=None  accumulatedSwitchingLosses=0 J
  PS-Simulink Converter : nesl_utility/PS-Simulink Converter  PhysicalDomain=network_engine_domain  SubClassName=ps_output  LeftPortType=input  RightPortType=output  PseudoPeriodic=off  Frequencies=[]  VectorFormat=inherit  Unit=inherit  AffineConversion=off
  PS-Simulink Converter1 : nesl_utility/PS-Simulink Converter  PhysicalDomain=network_engine_domain  SubClassName=ps_output  LeftPortType=input  RightPortType=output  PseudoPeriodic=off  Frequencies=[]  VectorFormat=inherit  Unit=inherit  AffineConversion=off
  PWM Generator (DC-DC) : spsPWMGeneratorDCDCLib/PWM Generator (DC-DC)  Fsw=3000  Ts=5e-5
  Scope : Scope
  Scope1 : Scope
  Simulink-PS Converter : nesl_utility/Simulink-PS Converter  PhysicalDomain=network_engine_domain  SubClassName=ps_input  LeftPortType=input  RightPortType=output  PseudoPeriodic=off  Frequencies=[]  NoiseDistribution=none  NoiseParameters=[]  Unit=1  AffineConversion=off  FilteringAndDerivatives=provide  SimscapeFilterOrder=1  InputFilterTimeConstant=0.001  UdotUserProvided=0
  Simulink-PS Converter1 : nesl_utility/Simulink-PS Converter  PhysicalDomain=network_engine_domain  SubClassName=ps_input  LeftPortType=input  RightPortType=output  PseudoPeriodic=off  Frequencies=[]  NoiseDistribution=none  NoiseParameters=[]  Unit=1  AffineConversion=off  FilteringAndDerivatives=provide  SimscapeFilterOrder=1  InputFilterTimeConstant=0.001  UdotUserProvided=0
  Voltage Sensor : fl_lib/Electrical/Electrical Sensors/Voltage Sensor
  Voltage Sensor1 : fl_lib/Electrical/Electrical Sensors/Voltage Sensor
  + : PMIOPort  Side=Right
  - : PMIOPort  Port=2  Side=Right
  wires:
  PWM Generator (DC-DC)/1 -> Logical Operator/1, Simulink-PS Converter/1
  PS-Simulink Converter/1 -> Scope1/1
  PS-Simulink Converter1/1 -> Scope/1
  Logical Operator/1 -> Data Type Conversion/1
  Data Type Conversion/1 -> Simulink-PS Converter1/1
  U/1 -> PWM Generator (DC-DC)/1
  connections:
  "MOSFET (Ideal, Switching)1"/RConn2 -- Capacitor/RConn1 -- -/RConn1 -- Voltage Sensor1/RConn2 -- DC Voltage Source/RConn1 -- Voltage Sensor/RConn2
  "MOSFET (Ideal, Switching)"/RConn2 -- Inductor/LConn1 -- "MOSFET (Ideal, Switching)1"/RConn1
  DC Voltage Source/LConn1 -- "MOSFET (Ideal, Switching)"/RConn1 -- Voltage Sensor/LConn1
  Inductor/RConn1 -- Capacitor/LConn1 -- Voltage Sensor1/LConn1 -- +/RConn1
  Voltage Sensor/RConn1 -- PS-Simulink Converter/LConn1
  Voltage Sensor1/RConn1 -- PS-Simulink Converter1/LConn1
  Simulink-PS Converter/RConn1 -- "MOSFET (Ideal, Switching)"/LConn1
  Simulink-PS Converter1/RConn1 -- "MOSFET (Ideal, Switching)1"/LConn1

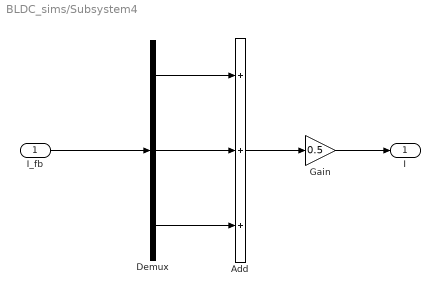
== system BLDC_sims/Subsystem4 ==
  I_fb : Inport
  Add : Sum  Inputs=+++
  Demux : Demux  Outputs=3
  Gain : Gain  Gain=0.5
  I : Outport
  wires:
  Demux/1 -> Add/1
  Demux/3 -> Add/3
  Demux/2 -> Add/2
  Add/1 -> Gain/1
  Gain/1 -> I/1
  I_fb/1 -> Demux/1

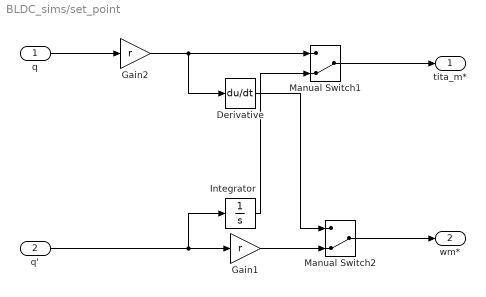
== system BLDC_sims/set_point ==
  q : Inport
  q' : Inport  Port=2
  Derivative : Derivative
  Gain1 : Gain  Gain=r
  Gain2 : Gain  Gain=r
  Integrator : Integrator
  Manual Switch1 : ManualSwitch  CurrentSetting=0
  Manual Switch2 : ManualSwitch  CurrentSetting=0
  tita_m* : Outport
  wm* : Outport  Port=2
  wires:
  Gain2/1 -> Manual Switch1/1, Derivative/1
  Manual Switch1/1 -> tita_m*/1
  q/1 -> Gain2/1
  Derivative/1 -> Manual Switch2/1
  q'/1 -> Integrator/1, Gain1/1
  Manual Switch2/1 -> wm*/1
  Integrator/1 -> Manual Switch1/2
  Gain1/1 -> Manual Switch2/2
